simulink model "EvitarPared"  (R2023b)
settings: Solver=VariableStepAuto  StartTime=0.0  StopTime=10.0  RelTol=1e-3
libraries: simulink x4
settings Model: Creator=Usuario_UMA  LastModifiedBy=Usuario

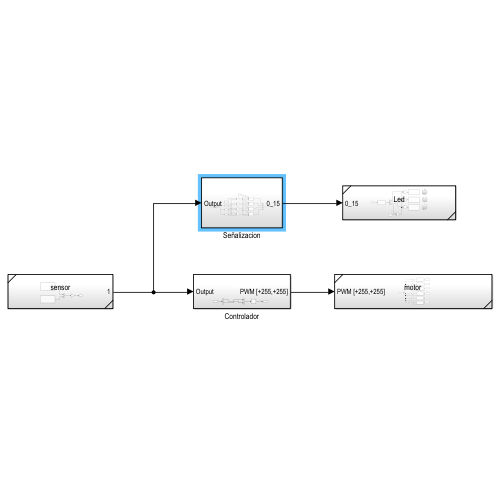
[thumbnail: Simulink's stored preview of the top-level diagram]
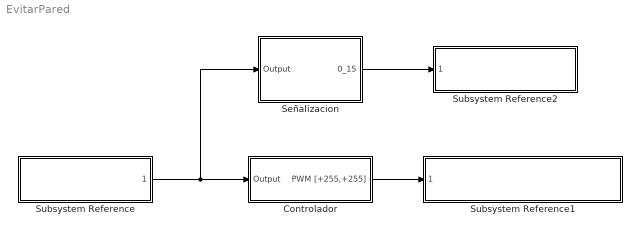
== system EvitarPared ==
  Controlador : Subsystem
  Señalizacion : Subsystem
  Subsystem Reference : Subsystem  ReferencedSubsystem=sensor
  Subsystem Reference1 : Subsystem  ReferencedSubsystem=motor
  Subsystem Reference2 : Subsystem  ReferencedSubsystem=Led
  wires:
  Subsystem Reference/1 -> Señalizacion/1(Output), Controlador/1(Output)
  Controlador/1(PWM [+255,+255]) -> Subsystem Reference1/1
  Señalizacion/1(0_15) -> Subsystem Reference2/1

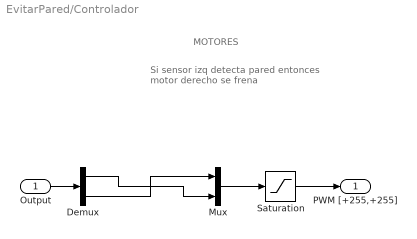
== system EvitarPared/Controlador ==
  note: MOTORES
  note: Si sensor izq detecta pared entonces motor derecho se frena
  Output : Inport
  Demux : Demux  Outputs=2
  Mux : Mux  Inputs=2
  Saturation : Saturate
  PWM [+255,+255] : Outport
  wires:
  Output/1 -> Demux/1
  Demux/2 -> Mux/1
  Mux/1 -> Saturation/1
  Saturation/1 -> PWM [+255,+255]/1
  Demux/1 -> Mux/2

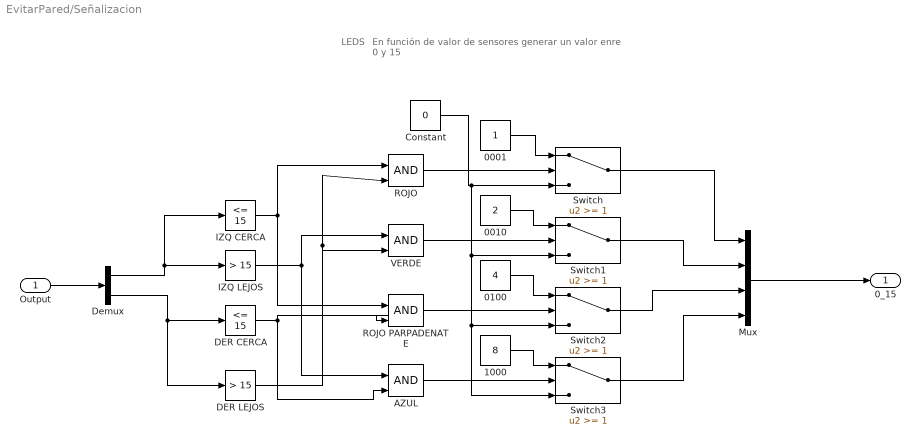
== system EvitarPared/Señalizacion ==
  note: En función de valor de sensores generar un valor enre 0 y 15
  note: LEDS
  Output : Inport
  0001 : Constant
  0010 : Constant  Value=2
  0100 : Constant  Value=4
  1000 : Constant  Value=8
  AZUL : Logic  IconShape=distinctive  AllPortsSameDT=off  OutDataTypeStr=boolean
  Constant : Constant  Value=0
  DER CERCA : simulink/Logic and Bit Operations/Compare To Constant  relop=<=  const=15  OutDataTypeStr=boolean
  "DER LEJOS " : simulink/Logic and Bit Operations/Compare To Constant  relop=>  const=15  OutDataTypeStr=boolean
  Demux : Demux  Outputs=2
  IZQ CERCA : simulink/Logic and Bit Operations/Compare To Constant  relop=<=  const=15  OutDataTypeStr=boolean
  IZQ LEJOS : simulink/Logic and Bit Operations/Compare To Constant  relop=>  const=15  OutDataTypeStr=boolean
  Mux : Mux
  ROJO : Logic  IconShape=distinctive  AllPortsSameDT=off  OutDataTypeStr=boolean
  ROJO PARPADENATE : Logic  IconShape=distinctive  AllPortsSameDT=off  OutDataTypeStr=boolean
  Switch{,1..3} (4 alike) : Switch  Threshold=1  OutDataTypeStr=int8  SaturateOnIntegerOverflow=off  InputSameDT=off
  VERDE : Logic  IconShape=distinctive  AllPortsSameDT=off  OutDataTypeStr=boolean
  0_15 : Outport
  wires:
  Output/1 -> Demux/1
  Mux/1 -> 0_15/1
  Demux/1 -> IZQ CERCA/1, IZQ LEJOS/1
  Demux/2 -> "DER LEJOS "/1, DER CERCA/1
  IZQ CERCA/1 -> ROJO PARPADENATE/1, ROJO/1
  "DER LEJOS "/1 -> ROJO/2, VERDE/2
  IZQ LEJOS/1 -> VERDE/1, AZUL/1
  DER CERCA/1 -> ROJO PARPADENATE/2, AZUL/2
  ROJO/1 -> Switch/2
  VERDE/1 -> Switch1/2
  ROJO PARPADENATE/1 -> Switch2/2
  AZUL/1 -> Switch3/2
  Constant/1 -> Switch/3, Switch1/3, Switch2/3, Switch3/3
  0010/1 -> Switch1/1
  0100/1 -> Switch2/1
  1000/1 -> Switch3/1
  0001/1 -> Switch/1
  Switch3/1 -> Mux/4
  Switch2/1 -> Mux/3
  Switch1/1 -> Mux/2
  Switch/1 -> Mux/1
